simulink model "SARLsimulink2"  (R2023a)
settings: Solver=VariableStepAuto  StartTime=0.0  StopTime=10.0  RelTol=1e-3
settings Model: Creator=Ethan  LastModifiedBy=Ethan

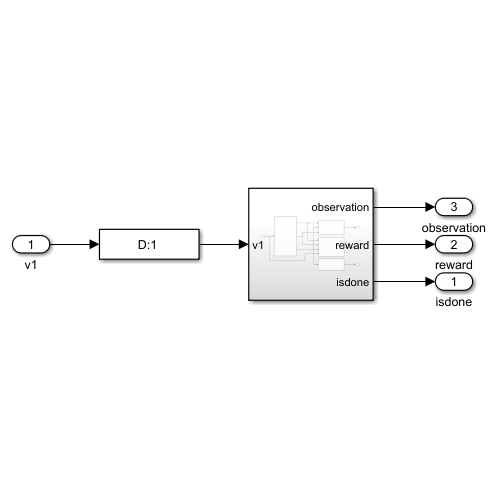
[thumbnail: Simulink's stored preview of the top-level diagram]
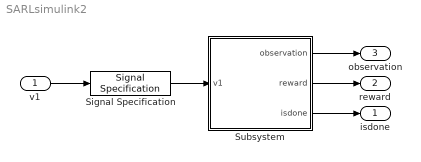
== system SARLsimulink2 ==
  v1 : Inport
  Signal Specification : SignalSpecification  Dimensions=1
  Subsystem : Subsystem
  isdone : Outport
  reward : Outport  Port=2
  observation : Outport  Port=3
  wires:
  v1/1 -> Signal Specification/1
  Subsystem/3(isdone) -> isdone/1
  Subsystem/1(observation) -> observation/1
  Signal Specification/1 -> Subsystem/1(v1)
  Subsystem/2(reward) -> reward/1

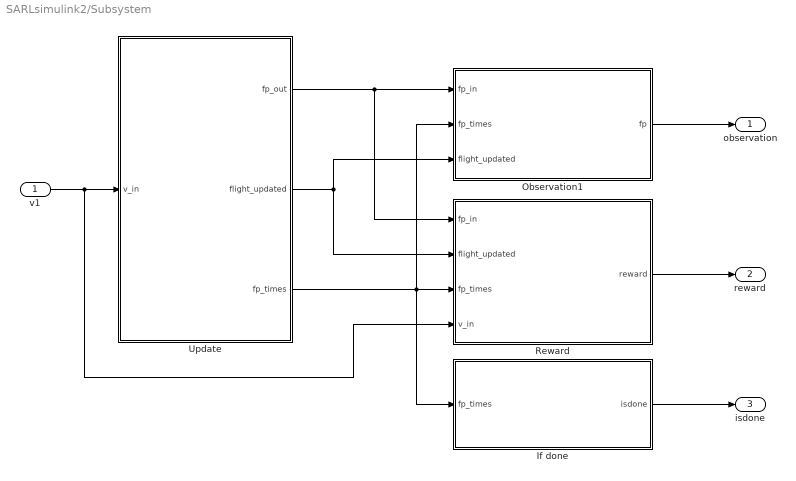
== system SARLsimulink2/Subsystem ==
  v1 : Inport
  If done : MATLAB Function  TreatAsAtomicUnit=on
  Observation1 : Subsystem
  Reward : MATLAB Function  TreatAsAtomicUnit=on
  Update : MATLAB Function  TreatAsAtomicUnit=on
  observation : Outport
  reward : Outport  Port=2
  isdone : Outport  Port=3
  wires:
  Update/1(fp_out) -> Reward/1(fp_in), Observation1/1(fp_in)
  v1/1 -> Reward/4(v_in), Update/1(v_in)
  Reward/1(reward) -> reward/1
  Update/3(fp_times) -> If done/1(fp_times), Observation1/2(fp_times), Reward/3(fp_times)
  Update/2(flight_updated) -> Reward/2(flight_updated), Observation1/3(flight_updated)
  If done/1(isdone) -> isdone/1
  Observation1/1(fp) -> observation/1

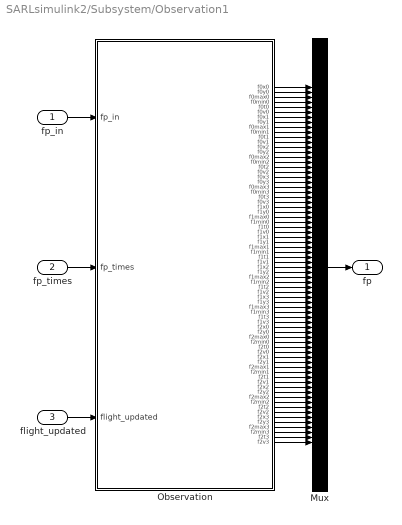
== system SARLsimulink2/Subsystem/Observation1 ==
  fp_in : Inport
  fp_times : Inport  Port=2
  flight_updated : Inport  Port=3
  Mux : Mux  Inputs=72
  Observation : MATLAB Function  TreatAsAtomicUnit=on
  fp : Outport
  wires:
  fp_in/1 -> Observation/1(fp_in)
  fp_times/1 -> Observation/2(fp_times)
  flight_updated/1 -> Observation/3(flight_updated)
  Mux/1 -> fp/1
  Observation/72(f2v3) -> Mux/72
  Observation/70(f2min3) -> Mux/70
  Observation/71(f2t3) -> Mux/71
  Observation/69(f2max3) -> Mux/69
  Observation/68(f2y3) -> Mux/68
  Observation/66(f2v2) -> Mux/66
  Observation/67(f2x3) -> Mux/67
  Observation/65(f2t2) -> Mux/65
  Observation/63(f2max2) -> Mux/63
  Observation/64(f2min2) -> Mux/64
  Observation/62(f2y2) -> Mux/62
  Observation/61(f2x2) -> Mux/61
  Observation/59(f2t1) -> Mux/59
  Observation/60(f2v1) -> Mux/60
  Observation/58(f2min1) -> Mux/58
  Observation/57(f2max1) -> Mux/57
  Observation/56(f2y1) -> Mux/56
  Observation/54(f2v0) -> Mux/54
  Observation/55(f2x1) -> Mux/55
  Observation/53(f2t0) -> Mux/53
  Observation/52(f2min0) -> Mux/52
  Observation/51(f2max0) -> Mux/51
  Observation/50(f2y0) -> Mux/50
  Observation/49(f2x0) -> Mux/49
  Observation/47(f1t3) -> Mux/47
  Observation/48(f1v3) -> Mux/48
  Observation/46(f1min3) -> Mux/46
  Observation/45(f1max3) -> Mux/45
  Observation/43(f1x3) -> Mux/43
  Observation/44(f1y3) -> Mux/44
  Observation/42(f1v2) -> Mux/42
  Observation/40(f1min2) -> Mux/40
  Observation/41(f1t2) -> Mux/41
  Observation/38(f1y2) -> Mux/38
  Observation/39(f1max2) -> Mux/39
  Observation/37(f1x2) -> Mux/37
  Observation/35(f1t1) -> Mux/35
  Observation/36(f1v1) -> Mux/36
  Observation/34(f1min1) -> Mux/34
  Observation/33(f1max1) -> Mux/33
  Observation/32(f1y1) -> Mux/32
  Observation/31(f1x1) -> Mux/31
  Observation/30(f1v0) -> Mux/30
  Observation/29(f1t0) -> Mux/29
  Observation/28(f1min0) -> Mux/28
  Observation/27(f1max0) -> Mux/27
  Observation/26(f1y0) -> Mux/26
  Observation/25(f1x0) -> Mux/25
  Observation/24(f0v3) -> Mux/24
  Observation/23(f0t3) -> Mux/23
  Observation/22(f0min3) -> Mux/22
  Observation/21(f0max3) -> Mux/21
  Observation/20(f0y3) -> Mux/20
  Observation/19(f0x3) -> Mux/19
  Observation/18(f0v2) -> Mux/18
  Observation/17(f0t2) -> Mux/17
  Observation/1(f0x0) -> Mux/1
  Observation/2(f0y0) -> Mux/2
  Observation/3(f0max0) -> Mux/3
  Observation/4(f0min0) -> Mux/4
  Observation/5(f0t0) -> Mux/5
  Observation/6(f0v0) -> Mux/6
  Observation/7(f0x1) -> Mux/7
  Observation/8(f0y1) -> Mux/8
  Observation/9(f0max1) -> Mux/9
  Observation/10(f0min1) -> Mux/10
  Observation/11(f0t1) -> Mux/11
  Observation/12(f0v1) -> Mux/12
  Observation/13(f0x2) -> Mux/13
  Observation/14(f0y2) -> Mux/14
  Observation/15(f0max2) -> Mux/15
  Observation/16(f0min2) -> Mux/16

== matlab function SARLsimulink2/Subsystem/If done ==
  data: fp_times input; isdone output
function isdone  = fcn(fp_times)

check = all(isnan(fp_times(:,1)));

if check
    isdone = 1;
else
    isdone = 0;
end

end

== matlab function SARLsimulink2/Subsystem/Observation1/Observation ==
  data: fp_in input; f0x0 output; fp_times input; flight_updated input; f0y0 output; f0max0 output; f0min0 output; f0t0 output; f0v0 output; f0x1 output; f0y1 output; f0max1 output; f0min1 output; f0t1 output; f0v1 output; f0x2 output; f0y2 output; f0max2 output; f0min2 output; f0t2 output; f0v2 output; f0x3 output; f0y3 output; f0max3 output; f0min3 output; f0t3 output; f0v3 output; f1x0 output; f1y0 output; f1max0 output; f1min0 output; f1t0 output; f1v0 output; f1x1 output; f1y1 output; f1max1 output; f1min1 output; f1t1 output; f1v1 output; f1x2 output; f1y2 output; f1max2 output; f1min2 output; f1t2 output; f1v2 output; f1x3 output; f1y3 output; f1max3 output; f1min3 output; f1t3 output; f1v3 output; f2x0 output; f2y0 output; f2max0 output; f2min0 output; f2t0 output; f2v0 output; f2x1 output; f2y1 output; f2max1 output; f2min1 output; f2t1 output; f2v1 output; f2x2 output; f2y2 output; f2max2 output; f2min2 output; f2t2 output; f2v2 output; f2x3 output; f2y3 output; f2max3 output; f2min3 output; f2t3 output; f2v3 output
function [f0x0,f0y0,f0max0,f0min0,f0t0,f0v0, f0x1,f0y1,f0max1,f0min1,f0t1,f0v1, f0x2,f0y2,f0max2,f0min2,f0t2,f0v2, f0x3,f0y3,f0max3,f0min3,f0t3,f0v3,  f1x0,f1y0,f1max0,f1min0,f1t0,f1v0, f1x1,f1y1,f1max1,f1min1,f1t1,f1v1, f1x2,f1y2,f1max2,f1min2,f1t2,f1v2, f1x3,f1y3,f1max3,f1min3,f1t3,f1v3,  f2x0,f2y0,f2max0,f2min0,f2t0,f2v0, f2x1,f2y1,f2max1,f2min1,f2t1,f2v1, f2x2,f2y2,f2max2,f2min2,f2t2,f2v2, f2x3,f2y3,f2max3,f2min3,f2t3,f2v3] = fcn(fp_in,fp_times,flight_updated)
    
    t1 = flight_updated(1,3);
    timebelow = 20;  

   
    col = [0];
    
    
    for i = 1:size(fp_times, 1)
        if ~isnan(fp_times(i, 1)) && (fp_times(i, 1) >= (t1 - timebelow) && fp_times(i, 1) <= t1)  % distance will be based on the lastest flight on the updated state
            col = [col; i];
        end
    end
    length_col = length(col);

        f0x0    = 0;
        f0y0    = 0;
        f0max0  = 0;
        f0min0  = 0;
        f0t0    = 0;
        f0v0    = 0;
        
        f0x1    = fp_in(flight_updated(1,2),(flight_updated(1,1)*6)-5);
        f0y1    = fp_in(flight_updated(1,2),(flight_updated(1,1)*6)-4);
        f0max1  = fp_in(flight_updated(1,2),(flight_updated(1,1)*6)-3);
        f0min1  = fp_in(flight_updated(1,2),(flight_updated(1,1)*6)-2);
        f0t1    = fp_in(flight_updated(1,2),(flight_updated(1,1)*6)-1);
        f0v1    = fp_in(flight_updated(1,2),(flight_updated(1,1)*6));

        f0x2    = fp_in(flight_updated(1,2)+1,(flight_updated(1,1)*6)-5);
        f0y2    = fp_in(flight_updated(1,2)+1,(flight_updated(1,1)*6)-4);
        f0max2  = fp_in(flight_updated(1,2)+1,(flight_updated(1,1)*6)-3);
        f0min2  = fp_in(flight_updated(1,2)+1,(flight_updated(1,1)*6)-2);
        f0t2    = fp_in(flight_updated(1,2)+1,(flight_updated(1,1)*6)-1);
        f0v2    = fp_in(flight_updated(1,2)+1,(flight_updated(1,1)*6));

        f0x3    = fp_in(flight_updated(1,2)+2,(flight_updated(1,1)*6)-5);
        f0y3    = fp_in(flight_updated(1,2)+2,(flight_updated(1,1)*6)-4);
        f0max3  = fp_in(flight_updated(1,2)+2,(flight_updated(1,1)*6)-3);
        f0min3  = fp_in(flight_updated(1,2)+2,(flight_updated(1,1)*6)-2);
        f0t3    = fp_in(flight_updated(1,2)+2,(flight_updated(1,1)*6)-1);
        f0v3    = fp_in(flight_updated(1,2)+2,(flight_updated(1,1)*6));

        
        f1x0    = 0;
        f1y0    = 0;
        f1max0  = 0;
        f1min0  = 0;
        f1t0    = 0;
        f1v0    = 0;

        f1x1    = 0;
        f1y1    = 0;
        f1max1  = 0;
        f1min1  = 0;
        f1t1    = 0;
        f1v1    = 0;

        f1x2    = 0;
        f1y2    = 0;
        f1max2  = 0;
        f1min2  = 0;
        f1t2    = 0;
        f1v2    = 0;

        f1x3    = 0;
        f1y3    = 0;
        f1max3  = 0;
        f1min3  = 0;
        f1t3    = 0;
        f1v3    = 0;

        
        f2x0    = 0;
        f2y0    = 0;
        f2max0  = 0;
        f2min0  = 0;
        f2t0    = 0;
        f2v0    = 0;
        
        f2x1    = 0;
        f2y1    = 0;
        f2max1  = 0;
        f2min1  = 0;
        f2t1    = 0;
        f2v1    = 0;

        f2x2    = 0;
        f2y2    = 0;
        f2max2  = 0;
        f2min2  = 0;
        f2t2    = 0;
        f2v2    = 0;

        f2x3    = 0;
        f2y3    = 0;
        f2max3  = 0;
        f2min3  = 0;
        f2t3    = 0;
        f2v3    = 0;

    %%
    if length(col) == 2
        col_numbers = zeros(length_col,2);
        col_numbers(1,1) = col(2,1)*6;                    
        col_numbers(1,2) = fp_times(col(2,1),3);                
        
        f1x0    = fp_in(col_numbers(1,2)-1,col_numbers(1,1)-5); 
        f1y0    = fp_in(col_numbers(1,2)-1,col_numbers(1,1)-4);
        f1max0  = fp_in(col_numbers(1,2)-1,col_numbers(1,1)-3);
        f1min0  = fp_in(col_numbers(1,2)-1,col_numbers(1,1)-2);
        f1t0    = fp_in(col_numbers(1,2)-1,col_numbers(1,1)-1);
        f1v0    = fp_in(col_numbers(1,2)-1,col_numbers(1,1));
        
        f1x1    = fp_in(col_numbers(1,2),col_numbers(1,1)-5); 
        f1y1    = fp_in(col_numbers(1,2),col_numbers(1,1)-4);
        f1max1  = fp_in(col_numbers(1,2),col_numbers(1,1)-3);
        f1min1  = fp_in(col_numbers(1,2),col_numbers(1,1)-2);
        f1t1    = fp_in(col_numbers(1,2),col_numbers(1,1)-1);
        f1v1    = fp_in(col_numbers(1,2),col_numbers(1,1));

        f1x2    = fp_in(col_numbers(1,2)+1,col_numbers(1,1)-5); 
        f1y2    = fp_in(col_numbers(1,2)+1,col_numbers(1,1)-4);
        f1max2  = fp_in(col_numbers(1,2)+1,col_numbers(1,1)-3);
        f1min2  = fp_in(col_numbers(1,2)+1,col_numbers(1,1)-2);
        f1t2    = fp_in(col_numbers(1,2)+1,col_numbers(1,1)-1);
        f1v2    = fp_in(col_numbers(1,2)+1,col_numbers(1,1));

        f1x3    = fp_in(col_numbers(1,2)+2,col_numbers(1,1)-5); 
        f1y3    = fp_in(col_numbers(1,2)+2,col_numbers(1,1)-4);
        f1max3  = fp_in(col_numbers(1,2)+2,col_numbers(1,1)-3);
        f1min3  = fp_in(col_numbers(1,2)+2,col_numbers(1,1)-2);
        f1t3    = fp_in(col_numbers(1,2)+2,col_numbers(1,1)-1);
        f1v3    = fp_in(col_numbers(1,2)+2,col_numbers(1,1));

    elseif length(col) >= 3
        col_numbers = zeros(length_col,2);
        col_numbers(1,1) = col(2,1)*6;                          
        col_numbers(1,2) = fp_times(col(2,1),3);             
        
        f1x0    = fp_in(col_numbers(1,2)-1,col_numbers(1,1)-5); 
        f1y0    = fp_in(col_numbers(1,2)-1,col_numbers(1,1)-4);
        f1max0  = fp_in(col_numbers(1,2)-1,col_numbers(1,1)-3);
        f1min0  = fp_in(col_numbers(1,2)-1,col_numbers(1,1)-2);
        f1t0    = fp_in(col_numbers(1,2)-1,col_numbers(1,1)-1);
        f1v0    = fp_in(col_numbers(1,2)-1,col_numbers(1,1));
        
        f1x1    = fp_in(col_numbers(1,2),col_numbers(1,1)-5); 
        f1y1    = fp_in(col_numbers(1,2),col_numbers(1,1)-4);
        f1max1  = fp_in(col_numbers(1,2),col_numbers(1,1)-3);
        f1min1  = fp_in(col_numbers(1,2),col_numbers(1,1)-2);
        f1t1    = fp_in(col_numbers(1,2),col_numbers(1,1)-1);
        f1v1    = fp_in(col_numbers(1,2),col_numbers(1,1));

        f1x2    = fp_in(col_numbers(1,2)+1,col_numbers(1,1)-5); 
        f1y2    = fp_in(col_numbers(1,2)+1,col_numbers(1,1)-4);
        f1max2  = fp_in(col_numbers(1,2)+1,col_numbers(1,1)-3);
        f1min2  = fp_in(col_numbers(1,2)+1,col_numbers(1,1)-2);
        f1t2    = fp_in(col_numbers(1,2)+1,col_numbers(1,1)-1);
        f1v2    = fp_in(col_numbers(1,2)+1,col_numbers(1,1));

        f1x3    = fp_in(col_numbers(1,2)+2,col_numbers(1,1)-5); 
        f1y3    = fp_in(col_numbers(1,2)+2,col_numbers(1,1)-4);
        f1max3  = fp_in(col_numbers(1,2)+2,col_numbers(1,1)-3);
        f1min3  = fp_in(col_numbers(1,2)+2,col_numbers(1,1)-2);
        f1t3    = fp_in(col_numbers(1,2)+2,col_numbers(1,1)-1);
        f1v3    = fp_in(col_numbers(1,2)+2,col_numbers(1,1));

        col_numbers(2,1) = col(3,1)*6;                         
        col_numbers(2,2) = fp_times(col(3,1),3);               
        
        f2x0    = fp_in(col_numbers(2,2)-1,col_numbers(2,1)-5); 
        f2y0    = fp_in(col_numbers(2,2)-1,col_numbers(2,1)-4);
        f2max0  = fp_in(col_numbers(2,2)-1,col_numbers(2,1)-3);
        f2min0  = fp_in(col_numbers(2,2)-1,col_numbers(2,1)-2);
        f2t0    = fp_in(col_numbers(2,2)-1,col_numbers(2,1)-1);
        f2v0    = fp_in(col_numbers(2,2)-1,col_numbers(2,1));
        
        f2x1    = fp_in(col_numbers(2,2),col_numbers(2,1)-5); 
        f2y1    = fp_in(col_numbers(2,2),col_numbers(2,1)-4);
        f2max1  = fp_in(col_numbers(2,2),col_numbers(2,1)-3);
        f2min1  = fp_in(col_numbers(2,2),col_numbers(2,1)-2);
        f2t1    = fp_in(col_numbers(2,2),col_numbers(2,1)-1);
        f2v1    = fp_in(col_numbers(2,2),col_numbers(2,1));

        f2x2    = fp_in(col_numbers(2,2)+1,col_numbers(2,1)-5); 
        f2y2    = fp_in(col_numbers(2,2)+1,col_numbers(2,1)-4);
        f2max2  = fp_in(col_numbers(2,2)+1,col_numbers(2,1)-3);
        f2min2  = fp_in(col_numbers(2,2)+1,col_numbers(2,1)-2);
        f2t2    = fp_in(col_numbers(2,2)+1,col_numbers(2,1)-1);
        f2v2    = fp_in(col_numbers(2,2)+1,col_numbers(2,1));

        f2x3    = fp_in(col_numbers(2,2)+2,col_numbers(2,1)-5); 
        f2y3    = fp_in(col_numbers(2,2)+2,col_numbers(2,1)-4);
        f2max3  = fp_in(col_numbers(2,2)+2,col_numbers(2,1)-3);
        f2min3  = fp_in(col_numbers(2,2)+2,col_numbers(2,1)-2);
        f2t3    = fp_in(col_numbers(2,2)+2,col_numbers(2,1)-1);
        f2v3    = fp_in(col_numbers(2,2)+2,col_numbers(2,1));
    end

end

== matlab function SARLsimulink2/Subsystem/Update ==
  data: v_in input; fp_out output; flight_updated output; fp_times output; fp_in parameter
function [fp_out,flight_updated,fp_times]= fcn(v_in, fp_in)


%%

num_col = length(fp_in);     
int_col = round(num_col/6); 
fp_times = zeros(int_col,3);


if fp_in(2,5*1) == 0                         
    fp_times(1,1) = fp_in(1,5*1);
    fp_times(1,2) = fp_in(1,6*1);
    fp_times(1,3) = 1;
else
    fp1row = 3;
    while fp1row <= length(fp_in(:,1*1))
        if fp_in(fp1row,5*1) == 0
            if fp_in(fp1row-1,1*1) == 0 && fp_in(fp1row-1,2*1) == 0
                fp_times(1,1) = nan;
                fp_times(1,2) = nan;
                fp_times(1,3) = nan;
                break;
            else
                fp_times(1,1) = fp_in(fp1row-1,5*1);
                fp_times(1,2) = fp_in(fp1row-1,6*1);
                fp_times(1,3) = fp1row-1;
                break;
            end
        else
            fp_times(1,1) = nan;
        end
        fp1row = fp1row+1;
    end
end

for i = 2:length(fp_times)
    current_col = 6*(i-1);
    if fp_in(2,5+current_col) == 0                           
        fp_times(i,1) = fp_in(1,5+current_col);
        fp_times(i,2) = fp_in(1,6+current_col);
        fp_times(i,3) = 1;
    else
        fprow = 3;
        while fprow <= length(fp_in(:,1*i))
            if fp_in(fprow,5+current_col) == 0
                if fp_in(fprow-1,1+current_col) == 0 && fp_in(fprow-1,2+current_col) == 0
                    fp_times(i,1) = nan;
                    fp_times(i,2) = nan;
                    fp_times(i,3) = nan;
                    break;
                else
                    fp_times(i,1) = fp_in(fprow-1,5+current_col);
                    fp_times(i,2) = fp_in(fprow-1,6+current_col);
                    fp_times(i,3) = fprow-1;
                    break;
                end
            else
                fp_times(i,1) = nan;
            end
            fprow = fprow+1;
        end
    end
end

%% 

int_val = inf;
flight_number = 0;
for i = 1:length(fp_times)
    if isnan(fp_times(i,1))
        continue;
    end
    if fp_times(i,1) < int_val
        int_val = fp_times(i,1);
        flight_number = i;
    end
end

rowinfile = fp_times(flight_number,3);

%% UPDATE
  
current = flight_number*6;

v0 = fp_in(rowinfile,current);
v1 = (v_in+v0)*0.514444;          
t1 = NaN;
    if v1 <= 180*0.514444
        fp_in(rowinfile+1,current-1) = NaN;
        fp_in(rowinfile+1,current)   = NaN;
    else
        x0 = fp_in(rowinfile,current-5);
        x1 = fp_in(rowinfile+1,current-5);
        
        y0 = fp_in(rowinfile,current-4);
        y1 = fp_in(rowinfile+1,current-4);
        
        mag = sqrt((x1-x0)^2 + (y1-y0)^2);
        
        t0 = fp_in(rowinfile,current-1);
        
        t1 = t0 + (mag / v1);    
        
        
        fp_in(rowinfile+1,current-1) = t1;
        fp_in(rowinfile+1,current) = v1/0.514444;   
    end

fp_out = fp_in;    
flight_updated = [flight_number rowinfile+1 t1 v1/0.514444];
    


    %% OBSERVATION 
    %% 
    num_col = length(fp_in);
    int_col = round(num_col/6);
    fp_times = zeros(int_col,3);
    
   
    if fp_in(2,5*1) == 0                            
        fp_times(1,1) = fp_in(1,5*1);
        fp_times(1,2) = fp_in(1,6*1);
        fp_times(1,3) = 1;
    else
        fp1row = 3;
        while fp1row <= length(fp_in(:,1*1))
            if fp_in(fp1row,5*1) == 0
                if fp_in(fp1row-1,1*1) == 0 && fp_in(fp1row-1,2*1) == 0
                    fp_times(1,1) = nan;
                    fp_times(1,2) = nan;
                    fp_times(1,3) = nan;
                    break;
                else
                    fp_times(1,1) = fp_in(fp1row-1,5*1);
                    fp_times(1,2) = fp_in(fp1row-1,6*1);
                    fp_times(1,3) = fp1row-1;
                    break;
                end
            else
                fp_times(1,1) = nan;
            end
            fp1row = fp1row+1;
        end
    end
    
    for i = 2:length(fp_times)
        current_col = 6*(i-1);
        if fp_in(2,5+current_col) == 0                        
            fp_times(i,1) = fp_in(1,5+current_col);
            fp_times(i,2) = fp_in(1,6+current_col);
            fp_times(i,3) = 1;
        else
            fprow = 3;
            while fprow <= length(fp_in(:,1*i))
                if fp_in(fprow,5+current_col) == 0
                    if fp_in(fprow-1,1+current_col) == 0 && fp_in(fprow-1,2+current_col) == 0
                        fp_times(i,1) = nan;
                        fp_times(i,2) = nan;
                        fp_times(i,3) = nan;
                        break;
                    else
                        fp_times(i,1) = fp_in(fprow-1,5+current_col);
                        fp_times(i,2) = fp_in(fprow-1,6+current_col);
                        fp_times(i,3) = fprow-1;
                        break;
                    end
                else
                    fp_times(i,1) = nan;
                end
                fprow = fprow+1;
            end
        end
    end
    
end

== matlab function SARLsimulink2/Subsystem/Reward ==
  data: fp_in input; reward output; flight_updated input; fp_times input; v_in input
function reward    = fcn(fp_in,flight_updated,fp_times,v_in)


colinfile = flight_updated(1,1);     
currentflight = colinfile*6;
rowinfile = flight_updated(1,2);    
t1 = flight_updated(1,3);
v1 = flight_updated(1,4);          


%% For IAS change

if v_in ~= 0
    v_change = 0.0001;
    
else
    v_change = -0.00001;
end   

%% For max IAS and positive reward for completing a flight

v_max = fp_in(rowinfile,currentflight-3)/0.514444; % convert from m/s to knots


if v1 > v_max
    v_above = 0.000001*(v1-v_max);
    
else
    v_above = 0;
end



v_max = v_above;



%% For separation distance and congestion


timebelow = 20; 


col = [0];


for i = 1:size(fp_times, 1)
    if ~isnan(fp_times(i, 1)) && (fp_times(i, 1) <= (t1 - timebelow) && fp_times(i, 1) >= t1)  % distance will be based on the lastest flight on the updated state
        col = [col; i];
    end
end

x_current = fp_in(rowinfile,currentflight-5);
y_current = fp_in(rowinfile,currentflight-4);

length_col = length(col);



sep_25nm = 1852 * 2.5;
sep_5nm = 1852 * 7;    
sep_10nm = 1852 * 10;   
sep_20nm = 1852 * 20;  

if length_col == 1
    R_separation = 0;
    R_congestion = 0;
elseif length_col == 2
    col_numbers = zeros(length_col,4);
    col_numbers(1,1) = col(2,1)*6;                          
    col_numbers(1,2) = fp_times(col_numbers(1,1)/6,3);      
    col_numbers(1,3) = fp_in(col_numbers(1,2),col_numbers(1,1)-5);       
    col_numbers(1,4) = fp_in(col_numbers(1,2),col_numbers(1,1)-4);      
    if (col_numbers(1,3) >= x_current-sep_25nm && col_numbers(1,3) <= x_current+sep_25nm) && (col_numbers(1,4) >= y_current-sep_25nm && col_numbers(1,4) <= y_current+sep_25nm)
        R_separation = 1;               
        
    elseif (col_numbers(1,3) >= x_current-sep_5nm && col_numbers(1,3) <= x_current+sep_5nm) && (col_numbers(1,4) >= y_current-sep_5nm && col_numbers(1,4) <= y_current+sep_5nm)
        R_separation = 0.5;             
        
    else
        R_separation = 0;
    end
    R_congestion = 0;

else
    col_numbers = zeros(length_col-1,4);
    for i = 2:length_col
        col_numbers(i-1,1) = col(i,1)*6;                          
        col_numbers(i-1,2) = fp_times(col_numbers(i-1,1)/6,3);  
        col_numbers(i-1,3) = fp_in((col_numbers(i-1,2)),col_numbers(i-1,1)-5);       
        col_numbers(i-1,4) = fp_in((col_numbers(i-1,2)),col_numbers(i-1,1)-4);      
    end


    i = 1;
    R_separation = 0;
    R_congestion = 0;
    while i <=length(col_numbers)
        if (col_numbers(i,3) >= x_current-sep_25nm && col_numbers(i,3) <= x_current+sep_25nm) && (col_numbers(i,4) >= y_current-sep_25nm && col_numbers(i,4) <= y_current+sep_25nm)
            R_separation = R_separation + 1;            
            
        elseif (col_numbers(i,3) >= x_current-sep_5nm && col_numbers(i,3) <= x_current+sep_5nm) && (col_numbers(i,4) >= y_current-sep_5nm && col_numbers(i,4) <= y_current+sep_5nm)
            R_separation = R_separation + 0.5;            
            
        else
            R_separation = R_separation + 0;
        end
        i = i + 1;
    end

    i = 1;
    while i <= length(col_numbers)
        if (col_numbers(i,3) >= x_current-sep_10nm && col_numbers(i,3) <= x_current+sep_10nm) && (col_numbers(i,4) >= y_current-sep_10nm && col_numbers(i,4) <= y_current+sep_10nm)
            R_congestion = R_congestion + 0.0001;              
            
        else
            R_congestion = R_congestion + 0;
        end
        i = i + 1;
    end

    i = 1;
    while i <= length(col_numbers)
        if (col_numbers(i,3) >= x_current-sep_20nm && col_numbers(i,3) <= x_current+sep_20nm) && (col_numbers(i,4) >= y_current-sep_20nm && col_numbers(i,4) <= y_current+sep_20nm)
            R_congestion = R_congestion + 0.00005;               
            
        else
            R_congestion = R_congestion + 0;
        end
        i = i + 1;
    end

end    


%% Overall reward

reward = - R_separation - R_congestion - v_change - v_max ;


end
